simulink model "singlePhase_passiveRL"  (R2024b)
settings: Solver=VariableStepAuto  StartTime=0.0  StopTime=0.2  RelTol=1e-3
InitFcn:
  | % call the initialization file
  | predCurrCtrl_ini;
undefined symbols (not defined in the file or in its folder): Par
libraries: spsDCVoltageSourceLib x2, spsCurrentMeasurementLib x1, spsGroundLib x1, spsSeriesRLCBranchLib x1, spsThreeLevelBridgeLib x1, sps_lib x1
settings Model: Creator=PetrosK  LastModifiedBy=horak
settings DebuggingCC: UnderspecifiedInitializationDetection=Classic  MergeDetectMultiDrivingBlocksExec=none
settings ModelReferenceCC: PropagateSignalLabelsOutOfModel=off

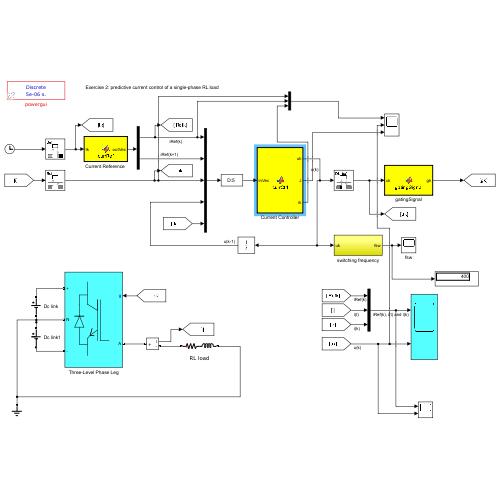
[thumbnail: Simulink's stored preview of the top-level diagram]
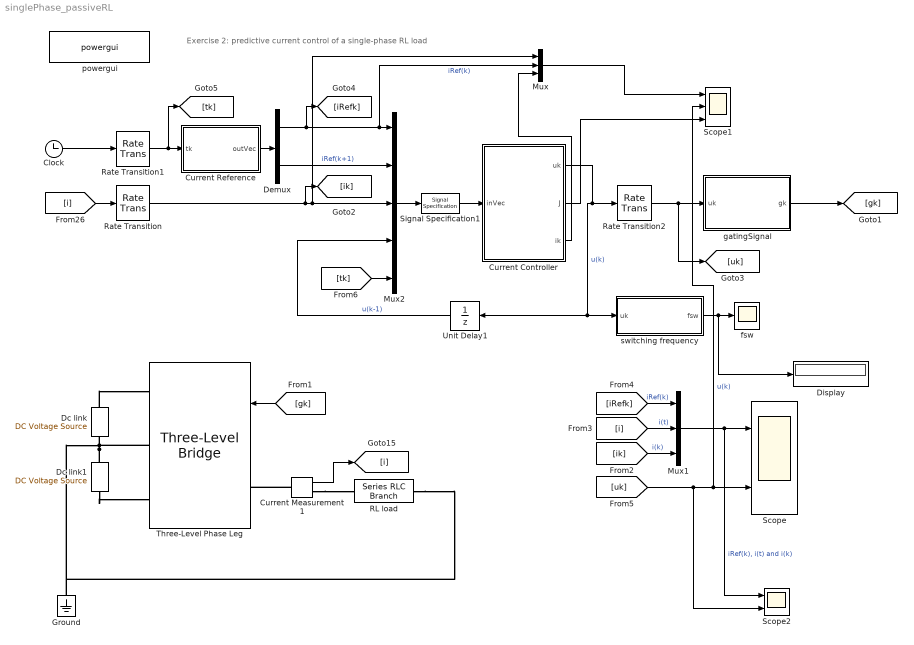
== system singlePhase_passiveRL ==
  note: Exercise 2: predictive current control of a single-phase RL load
  Clock : Clock
  Current Controller : MATLAB Function  TreatAsAtomicUnit=on
  Current Measurement1 : spsCurrentMeasurementLib/Current Measurement  PhasorSimulation=off  OutputType=Complex  PSBequivalent=0
  "Current Reference " : MATLAB Function  TreatAsAtomicUnit=on
  Dc link : spsDCVoltageSourceLib/DC Voltage Source  Amplitude=Par.SI.Vdc/2  Measurements=None
  Dc link1 : spsDCVoltageSourceLib/DC Voltage Source  Amplitude=Par.SI.Vdc/2  Measurements=None
  Demux : Demux  Outputs=2
  Display : Display
  Ground : spsGroundLib/Ground  LConnTagsString=a
  Mux : Mux  Inputs=3
  Mux1 : Mux  Inputs=3
  Mux2 : Mux  Inputs=5
  RL load : spsSeriesRLCBranchLib/Series RLC Branch  LConnTagsString=__new0  RConnTagsString=__new0  BranchType=RL  Resistance=Par.SI.R  Inductance=Par.SI.L  SetiL0=off  InitialCurrent=0  Capacitance=1e-6  Setx0=off  InitialVoltage=0  Measurements=None
  Rate Transition : RateTransition  Deterministic=off  OutPortSampleTime=Par.Ts.control
  Rate Transition1 : RateTransition  Deterministic=off  OutPortSampleTime=Par.Ts.control
  Rate Transition2 : RateTransition  Deterministic=off  OutPortSampleTime=Par.Ts.system
  Scope : Scope  NumInputPorts=2
  Scope1 : Scope  NumInputPorts=3
  Scope2 : Scope  NumInputPorts=2
  Signal Specification1 : SignalSpecification  Dimensions=5
  Three-Level Phase Leg : spsThreeLevelBridgeLib/Three-Level Bridge  Arms=1  SnubberResistance=1e5  SbubberCapacitance=inf  Device=IGBT / Diodes  Ron=1e-3  ForwardVoltages="[  0  0  ]"  Measurements=None
      settings: LibrarySourceBlock=sps_lib/Power Electronics/Three-Level Bridge
  Unit Delay1 : UnitDelay  SampleTime=-1  HasFrameUpgradeWarning=on
  fsw : Scope
  gatingSignal : MATLAB Function  TreatAsAtomicUnit=on
  powergui : sps_lib/powergui  Priority=1  SimulationMode=Discrete  SampleTime=Par.Ts.system  frequency=60  Iterations=50  frequencyindice=0  Pbase=100e6  ErrMax=1e-4  UnitsV=kV  UnitsW=MW  buscounter=0  FunctionMessages=off  echomessages=off  EnableUseOfTLC=off  CurrentSourceSwitches=off  DisableSnubberDevices=off  DisableRonSwitches=off  DisableVfSwitches=off  DisplayEquations=off  AutomaticDiscreteSolvers=off  SolverType=Tustin  Interpol=off  ExternalGateDelay=off  methode=off  Ts=0  x0status=zero  SPID=off  SwTol=0  HookPort=off  NonlinearTolerance=1e-4  nMaxIteration=100  ContinueOnMaxIteration=off  RestoreLinks=warning  ResistiveCurrentMeasurement=off  Frange=[0:2:500]  Ylog=off  Xlog=on  ShowGrid=off  save=off  variable=ZData  structure=0  ZoomFFT=off  StartTime=0.0  cycles=1  DisplayStyle=1  fundamental=60  FreqAxis=off  MaxFrequency=1000  frequencyindicesteady=1  RmsSteady=1  display=off
  switching frequency : Subsystem
  wires:
  Clock/1 -> Rate Transition1/1
  Rate Transition/1 -> Mux2/3, Mux/1, [ik]
  Current Measurement1/1 -> [i]
  [i] -> Rate Transition/1
  [gk] -> Three-Level Phase Leg/1
  Mux1/1 -> Scope2/1, Scope/1  "iRef(k), i(t) and i(k)"
  Rate Transition2/1 -> gatingSignal/1(uk), [uk]
  Current Controller/1(uk) -> switching frequency/1(uk), Unit Delay1/1, Rate Transition2/1  "u(k)"
  [i] -> Mux1/2  "i(t)"
  [iRefk] -> Mux1/1  "iRef(k)"
  Mux2/1 -> Signal Specification1/1
  [uk] -> Scope2/2, Scope1/2, Scope/2  "u(k)"
  Rate Transition1/1 -> [tk], "Current Reference "/1(tk)
  "Current Reference "/1(outVec) -> Demux/1
  switching frequency/1(fsw) -> Display/1, fsw/1
  Unit Delay1/1 -> Mux2/4  "u(k-1)"
  Demux/2 -> Mux2/2  "iRef(k+1)"
  Demux/1 -> [iRefk], Mux/2, Mux2/1  "iRef(k)"
  [ik] -> Mux1/3  "i(k)"
  [tk] -> Mux2/5
  Signal Specification1/1 -> Current Controller/1(inVec)
  gatingSignal/1(gk) -> [gk]
  Current Controller/2(J) -> Scope1/3
  Mux/1 -> Scope1/1
  Current Controller/3(ik) -> Mux/3
  connections:
  Dc link/LConn1 -- Dc link1/RConn1 -- RL load/RConn1 -- Ground/LConn1 -- Three-Level Phase Leg/RConn2
  Current Measurement1/LConn1 -- Three-Level Phase Leg/LConn1
  Current Measurement1/RConn1 -- RL load/LConn1
  Dc link/RConn1 -- Three-Level Phase Leg/RConn1
  Dc link1/LConn1 -- Three-Level Phase Leg/RConn3

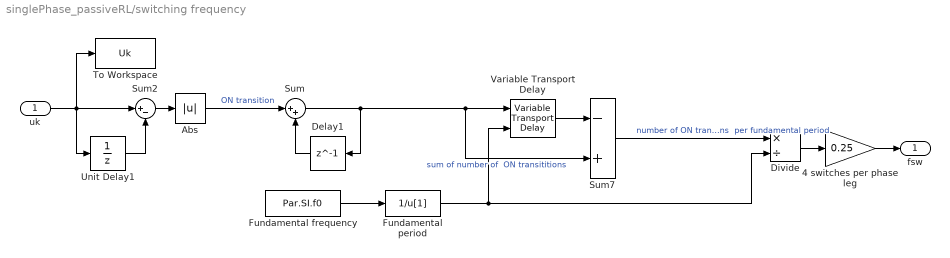
== system singlePhase_passiveRL/switching frequency ==
  uk : Inport
  4 switches per phase leg : Gain  Gain=0.25
  Abs : Abs  SaturateOnIntegerOverflow=off
  Delay1 : Delay  DelayLength=1  InitialCondition=0
  Divide : Product  Inputs=*/
  Fundamental frequency : Constant  Value=Par.SI.f0
  Fundamental period : Fcn  Expr=1/u[1]
  Sum : Sum  Inputs=|++
  Sum2 : Sum  Inputs=|+-
  Sum7 : Sum  Inputs=-+  InputSameDT=on  SaturateOnIntegerOverflow=on  OutDataTypeStr=Inherit: Same as first input
  To Workspace : ToWorkspace  VariableName=Uk  SaveFormat=Structure With Time  SampleTime=-1
  Unit Delay1 : UnitDelay  SampleTime=-1  HasFrameUpgradeWarning=on
  Variable Transport Delay : VariableTransportDelay  VariableDelayType=Variable transport delay  MaximumDelay=0.05  MaximumPoints=2048*4  PadeOrder=2
  fsw : Outport
  wires:
  Sum/1 -> Variable Transport Delay/1, Sum7/2, Delay1/1  "sum of number of  ON transititions"
  Variable Transport Delay/1 -> Sum7/1
  Delay1/1 -> Sum/2
  Fundamental frequency/1 -> Fundamental period/1
  Fundamental period/1 -> Divide/2, Variable Transport Delay/2
  Sum7/1 -> Divide/1  "number of ON transitions  per fundamental period"
  uk/1 -> To Workspace/1, Sum2/1, Unit Delay1/1
  Unit Delay1/1 -> Sum2/2
  Sum2/1 -> Abs/1
  Abs/1 -> Sum/1  "ON transition"
  Divide/1 -> 4 switches per phase leg/1
  4 switches per phase leg/1 -> fsw/1

== matlab function singlePhase_passiveRL/Current Controller ==
  data: inVec input; uk output; Par parameter; J output; ik output
function [uk, J,ik] = currCtrl(inVec, Par)

% Predictive current controller for a single-phase system with a 
% prediction horizon of one step
%
% Model Predictive Control of Power Electronic Systems, TAU, Tampere
% Petros Karamanakos, September 2025

% choose the controller 
contr = 'pred';         % 'hyst' or 'pred'

% interface
iRef_k = inVec(1);      % current reference at time step k
iRef_kp1 = inVec(2);    % current reference at time step k+1
ik = inVec(3);          % current sample at time step k
u_km1 = inVec(4);       % previous switch position applied at time step k-1
tk = inVec(5);          % actual time [s] - only for monitoring
 J=ones(1,3)*inf;
      

switch contr

    case 'hyst'
        %% simple three-level hysteresis controller

        iErr_thres = 100;      	% maximal tolerable current error [A]
        iErr = iRef_k - ik;     % actual current error

        % decision logic
        if iRef_k >= 0	% operation in the positive half-wave:
            % switch between 0 and 1
            if iErr > iErr_thres
                uk = 1;
            elseif iErr < -iErr_thres
                uk = 0;
            else
                uk = u_km1;
            end
        else         	% operation in the negative half-wave:
            % switch between -1 and 0
            if iErr > iErr_thres
                uk = 0;
            elseif iErr < -iErr_thres
                uk = -1;
            else
                uk = u_km1;
            end
        end

    case 'pred'
      all_uks={[0 -1],[1 0 -1],[0 1]};
      uks=all_uks{u_km1+2};
     
      for i=1:size(uks,2)
      
          ip=Par.Ctr.A*ik + Par.Ctr.B *uks(i) *Par.SI.Vdc/2;
          J(i)=((ip-iRef_kp1)/Par.Base.I)^2+Par.Ctr.lambda_u *abs(u_km1-uks(i));
           % J(i)=abs((ip-iRef_kp1)/Par.Base.I)+Par.Ctr.lambda_u *abs(u_km1-uks(i));
      end
      [~,index]=min(J);
      uk=uks(index);
    otherwise
        error('unknown control scheme');
end
J(J==inf)=0;
return

== matlab function singlePhase_passiveRL/Current Reference  ==
  data: tk input; outVec output; Par parameter
function outVec = currRef(tk, Par)

% Compute the current reference at time step k+1
%
% Model Predictive Control of Power Electronic Systems, TAU, Tampere
% Petros Karamanakos, September 2025

    m=0.8;

% current reference at time step k
iRef_k =m*Par.Base.I*sin(Par.Base.w*tk);

% current reference at time step k+1
iRef_kp1 =m* Par.Base.I*sin(Par.Base.w*(tk+Par.Ts.control));

% output interface
outVec = [iRef_k; iRef_kp1];

return

== matlab function singlePhase_passiveRL/gatingSignal ==
  data: uk input; gk output
function gk = gatingSignal(uk)

% Translate the switch position u(k) = {-1, 0, 1} into a gating signal for
% the 3-level phase leg g(k)
%
% Model Predictive Control of Power Electronic Systems, TAU, Tampere
% Petros Karamanakos, September 2025

vect={[0 0 1 1],[0 1 1 0],[1 1 0 0]};

gk=vect{uk+2};
return
